simulink model "robot_1"  (R2016a)
settings: Solver=ode1  StartTime=0.0  StopTime=1000  FixedStep=0.05  RelTol=1e-3
undefined symbols (not defined in the file): Angular, Linear
libraries: robotlib x4, realtime_pacer_lib x2, simulink x2
settings Model: Creator=Esther  LastModifiedBy=Esther
settings DataIOCC: LimitDataPoints=on  SaveFormat=Array
settings OptimizationCC: OptimizeModelRefInitCode=on  LifeSpan=1  MaxStackSize=64
settings HardwareCC: ProdBitPerPointer=32  ProdLargestAtomicFloat=None  ProdIntDivRoundTo=Undefined  ProdEndianess=Unspecified  ProdWordSize=32  ProdHWDeviceType=Generic->Unspecified (assume 32-bit Generic)
settings ModelReferenceCC: PropagateSignalLabelsOutOfModel=off
settings RTWCC: SystemTargetFile=ert.tlc  HardwareBoard=Robot Operating System (ROS)  PackageName=robot_1  TemplateMakefile=ert_default_tmf  Toolchain=Catkin  TargetLang=C++
settings ERTTargetCC: SupportContinuousTime=on  SupportVariableSizeSignals=on  RootIOFormat=Structure reference  ConvertIfToSwitch=off  SuppressUnreachableDefaultCases=off
settings ConfigComp: CovModelRefEnable=Off

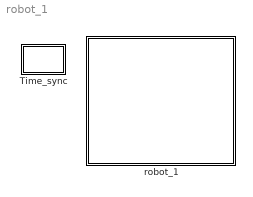
== system robot_1 ==
  Time_sync : Subsystem
  robot_1 : Subsystem

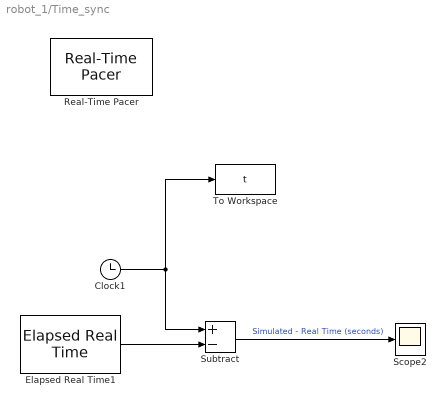
== system robot_1/Time_sync ==
  Clock1 : Clock
  Elapsed Real Time1 : realtime_pacer_lib/Elapsed Real Time
  Real-Time Pacer : realtime_pacer_lib/Real-Time Pacer  simTimePerRealTime=1
  Scope2 : Scope
  Subtract : Sum  Inputs=+-
  To Workspace : ToWorkspace  VariableName=t  SampleTime=-1
  wires:
  Elapsed Real Time1/1 -> Subtract/2
  Subtract/1 -> Scope2/1  "Simulated - Real Time (seconds)"
  Clock1/1 -> To Workspace/1, Subtract/1

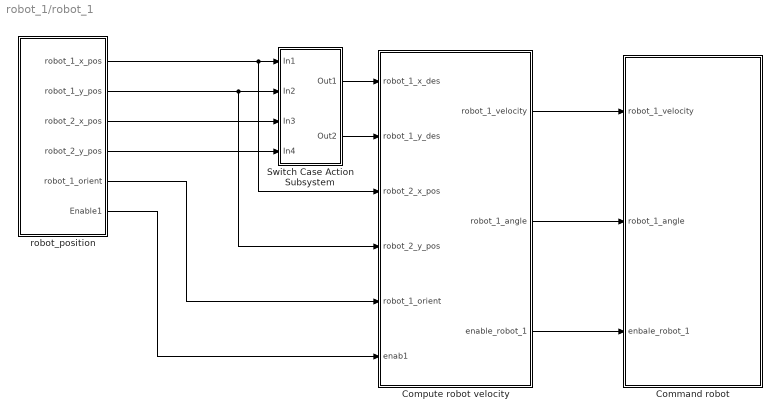
== system robot_1/robot_1 ==
  Command robot : Subsystem
  Compute robot velocity : Subsystem
  Switch Case Action Subsystem : Subsystem  TreatAsAtomicUnit=on
  robot_position : Subsystem
  wires:
  Compute robot velocity/1(robot_1_velocity) -> Command robot/1(robot_1_velocity)
  Compute robot velocity/3(enable_robot_1) -> Command robot/3(enbale_robot_1)
  robot_position/6(Enable1) -> Compute robot velocity/6(enab1)
  Switch Case Action Subsystem/1(Out1) -> Compute robot velocity/1(robot_1_x_des)
  robot_position/3(robot_2_x_pos) -> Switch Case Action Subsystem/3(In3)
  Switch Case Action Subsystem/2(Out2) -> Compute robot velocity/2(robot_1_y_des)
  robot_position/4(robot_2_y_pos) -> Switch Case Action Subsystem/4(In4)
  Compute robot velocity/2(robot_1_angle) -> Command robot/2(robot_1_angle)
  robot_position/5(robot_1_orient) -> Compute robot velocity/5(robot_1_orient)
  robot_position/2(robot_1_y_pos) -> Compute robot velocity/4(robot_2_y_pos), Switch Case Action Subsystem/2(In2)
  robot_position/1(robot_1_x_pos) -> Compute robot velocity/3(robot_2_x_pos), Switch Case Action Subsystem/1(In1)

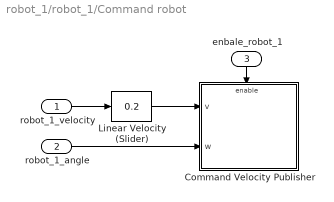
== system robot_1/robot_1/Command robot ==
  robot_1_velocity : Inport
  robot_1_angle : Inport  Port=2
  enbale_robot_1 : Inport  Port=3
  Command Velocity Publisher : Subsystem
  Linear Velocity (Slider) : simulink/Math Operations/Slider Gain  low=0  gain=0.2  high=1
  wires:
  robot_1_angle/1 -> Command Velocity Publisher/2(w)
  enbale_robot_1/1 -> Command Velocity Publisher/Enable
  robot_1_velocity/1 -> Linear Velocity (Slider)/1
  Linear Velocity (Slider)/1 -> Command Velocity Publisher/1(v)

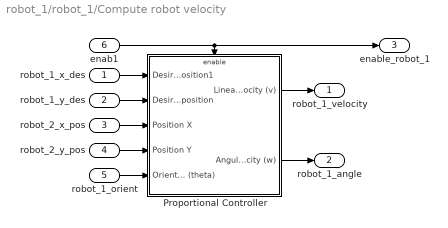
== system robot_1/robot_1/Compute robot velocity ==
  robot_1_x_des : Inport
  robot_1_y_des : Inport  Port=2
  robot_2_x_pos : Inport  Port=3
  robot_2_y_pos : Inport  Port=4
  robot_1_orient : Inport  Port=5
  enab1 : Inport  Port=6
  Proportional Controller : Subsystem
  robot_1_velocity : Outport
  robot_1_angle : Outport  Port=2
  enable_robot_1 : Outport  Port=3
  wires:
  Proportional Controller/1(Linear Velocity (v)) -> robot_1_velocity/1
  Proportional Controller/2(Angular Velocity (w)) -> robot_1_angle/1
  robot_2_x_pos/1 -> Proportional Controller/3(Position X)
  robot_1_orient/1 -> Proportional Controller/5(Orientation (theta))
  robot_1_x_des/1 -> Proportional Controller/1(Desired position1)
  robot_2_y_pos/1 -> Proportional Controller/4(Position Y)
  robot_1_y_des/1 -> Proportional Controller/2(Desired position)
  enab1/1 -> enable_robot_1/1, Proportional Controller/Enable

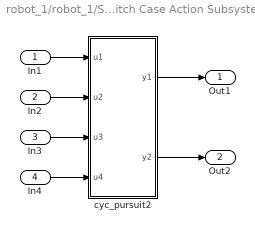
== system robot_1/robot_1/Switch Case Action Subsystem ==
  In1 : Inport
  In2 : Inport  Port=2
  In3 : Inport  Port=3
  In4 : Inport  Port=4
  cyc_pursuit2 : MATLAB Function  TreatAsAtomicUnit=on
  Out1 : Outport
  Out2 : Outport  Port=2
  wires:
  In4/1 -> cyc_pursuit2/4(u4)
  In3/1 -> cyc_pursuit2/3(u3)
  cyc_pursuit2/2(y2) -> Out2/1
  In2/1 -> cyc_pursuit2/2(u2)
  cyc_pursuit2/1(y1) -> Out1/1
  In1/1 -> cyc_pursuit2/1(u1)

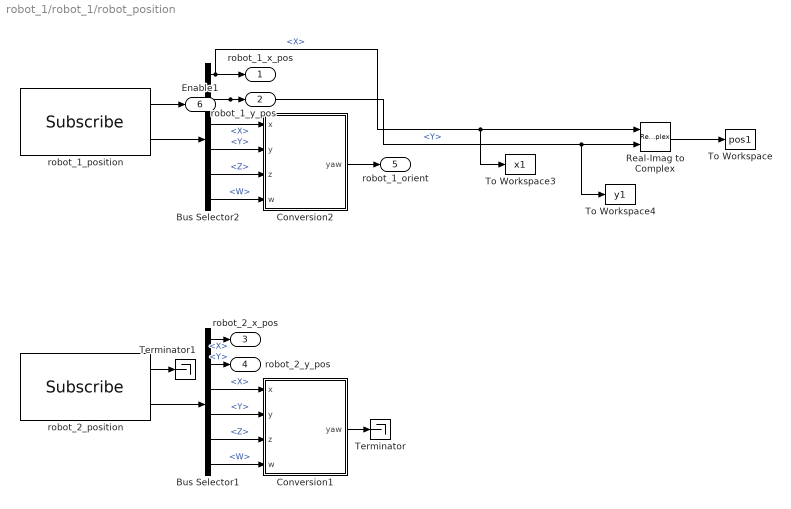
== system robot_1/robot_1/robot_position ==
  Bus Selector1 : BusSelector  OutputSignals=Pose.Pose.Position.X,Pose.Pose.Position.Y,Pose.Pose.Orientation.X,Pose.Pose.Orientation.Y,Pose.Pose.Orientation.Z,Pose.Pose.Orientation.W
  Bus Selector2 : BusSelector  OutputSignals=Pose.Pose.Position.X,Pose.Pose.Position.Y,Pose.Pose.Orientation.X,Pose.Pose.Orientation.Y,Pose.Pose.Orientation.Z,Pose.Pose.Orientation.W
  Conversion1 : MATLAB Function  TreatAsAtomicUnit=on
  Conversion2 : MATLAB Function  TreatAsAtomicUnit=on
  Real-Imag to Complex : RealImagToComplex
  Terminator : Terminator
  Terminator1 : Terminator
  To Workspace : ToWorkspace  VariableName=pos1  SampleTime=-1
  To Workspace3 : ToWorkspace  VariableName=x1  SampleTime=-1
  To Workspace4 : ToWorkspace  VariableName=y1  SampleTime=-1
  robot_1_position : robotlib/Subscribe  SourceLibraryInfo=This block requires Robotics System Toolbox  topicSource=Select from ROS network  topic=/robot_1/base_pose_ground_truth  messageType=nav_msgs/Odometry  sampleTime=-1  messageQueueLength=1
  robot_2_position : robotlib/Subscribe  SourceLibraryInfo=This block requires Robotics System Toolbox  topicSource=Select from ROS network  topic=/robot_2/base_pose_ground_truth  messageType=nav_msgs/Odometry  sampleTime=-1  messageQueueLength=1
  robot_1_x_pos : Outport
  robot_1_y_pos : Outport  Port=2
  robot_2_x_pos : Outport  Port=3
  robot_2_y_pos : Outport  Port=4
  robot_1_orient : Outport  Port=5
  Enable1 : Outport  Port=6
  wires:
  Bus Selector2/5 -> Conversion2/3(z)  "<Z>"
  robot_1_position/1 -> Enable1/1
  Bus Selector2/1 -> robot_1_x_pos/1, To Workspace3/1, Real-Imag to Complex/1  "<X>"
  Bus Selector2/4 -> Conversion2/2(y)  "<Y>"
  Bus Selector2/3 -> Conversion2/1(x)  "<X>"
  Real-Imag to Complex/1 -> To Workspace/1
  Bus Selector2/6 -> Conversion2/4(w)  "<W>"
  Bus Selector2/2 -> robot_1_y_pos/1, To Workspace4/1, Real-Imag to Complex/2  "<Y>"
  robot_1_position/2 -> Bus Selector2/1
  Conversion2/1(yaw) -> robot_1_orient/1
  Conversion1/1(yaw) -> Terminator/1
  Bus Selector1/1 -> robot_2_x_pos/1  "<X>"
  Bus Selector1/2 -> robot_2_y_pos/1  "<Y>"
  Bus Selector1/3 -> Conversion1/1(x)  "<X>"
  Bus Selector1/4 -> Conversion1/2(y)  "<Y>"
  Bus Selector1/5 -> Conversion1/3(z)  "<Z>"
  robot_2_position/2 -> Bus Selector1/1
  Bus Selector1/6 -> Conversion1/4(w)  "<W>"
  robot_2_position/1 -> Terminator1/1

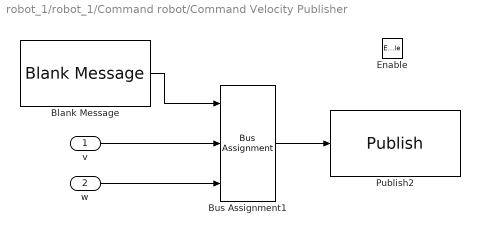
== system robot_1/robot_1/Command robot/Command Velocity Publisher ==
  v : Inport
  w : Inport  Port=2
  Enable : EnablePort
  Blank Message : robotlib/Blank Message  SourceLibraryInfo=This block requires Robotics System Toolbox  messageType=geometry_msgs/Twist  SampleTime=inf
  Bus Assignment1 : BusAssignment  DialogController=Simulink.DDGSource_BusAssignment  AssignedSignals=Linear.X,Angular.Z
  Publish2 : robotlib/Publish  SourceLibraryInfo=This block requires Robotics System Toolbox  topicSource=Select from ROS network  topic=/robot_1/cmd_vel  messageType=geometry_msgs/Twist  messageQueueLength=105
  wires:
  Bus Assignment1/1 -> Publish2/1
  Blank Message/1 -> Bus Assignment1/1
  v/1 -> Bus Assignment1/2
  w/1 -> Bus Assignment1/3

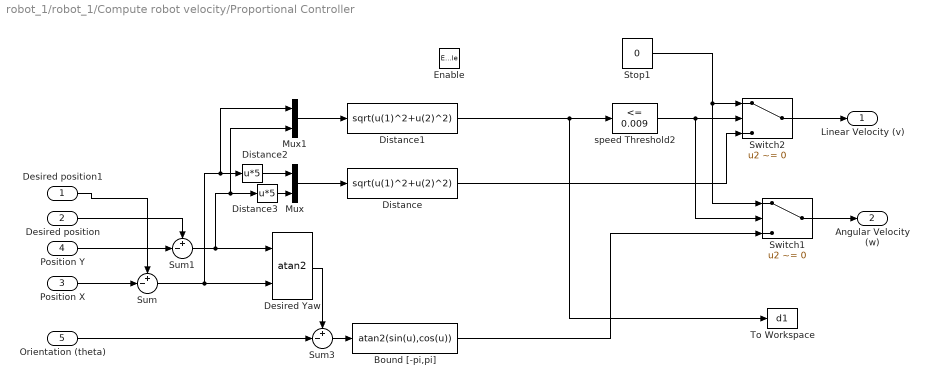
== system robot_1/robot_1/Compute robot velocity/Proportional Controller ==
  Desired position1 : Inport
  Desired position : Inport  Port=2
  Position X : Inport  Port=3
  Position Y : Inport  Port=4
  Orientation (theta) : Inport  Port=5
  Enable : EnablePort
  Bound [-pi,pi] : Fcn  Expr=atan2(sin(u),cos(u))
  Desired Yaw : Trigonometry  Operator=atan2
  Distance : Fcn  Expr=sqrt(u(1)^2+u(2)^2)
  Distance1 : Fcn  Expr=sqrt(u(1)^2+u(2)^2)
  Distance2 : Fcn  Expr=u*5
  Distance3 : Fcn  Expr=u*5
  Mux : Mux  Inputs=2
  Mux1 : Mux  Inputs=2
  Stop1 : Constant  Value=0
  Sum : Sum  Inputs=+-|
  Sum1 : Sum  Inputs=+-|
  Sum3 : Sum  Inputs=+-|
  Switch1 : Switch  Criteria=u2 ~= 0
  Switch2 : Switch  Criteria=u2 ~= 0
  To Workspace : ToWorkspace  VariableName=d1  SampleTime=-1
  speed Threshold2 : simulink/Logic and Bit Operations/Compare To Constant  relop=<=  const=0.009  OutDataTypeStr=boolean
  Linear Velocity (v) : Outport
  Angular Velocity (w) : Outport  Port=2
  wires:
  Desired position1/1 -> Sum/1
  Desired position/1 -> Sum1/1
  Position Y/1 -> Sum1/2
  Position X/1 -> Sum/2
  Mux/1 -> Distance/1
  Orientation (theta)/1 -> Sum3/2
  Desired Yaw/1 -> Sum3/1
  Sum3/1 -> Bound [-pi,pi]/1
  Distance/1 -> Switch2/3
  Distance2/1 -> Mux/1
  Distance3/1 -> Mux/2
  Mux1/1 -> Distance1/1
  Sum/1 -> Desired Yaw/2, Mux1/1, Distance2/1
  Sum1/1 -> Desired Yaw/1, Mux1/2, Distance3/1
  speed Threshold2/1 -> Switch2/2, Switch1/2
  Bound [-pi,pi]/1 -> Switch1/3
  Stop1/1 -> Switch2/1, Switch1/1
  Distance1/1 -> To Workspace/1, speed Threshold2/1
  Switch1/1 -> Angular Velocity (w)/1
  Switch2/1 -> Linear Velocity (v)/1

== matlab function robot_1/Switch Case Action Subsystem/cyc_pursuit2 ==
  data: u1 input; y1 output; u2 input; u3 input; u4 input; y2 output
function [y1, y2] = fcn(u1, u2, u3, u4)
%#codegen


y1 = ((1-0.2)*u1+(u3*0.2)-(2.5000*0.2));
y2 = ((1-0.2)*u2+(0.2*u4)-(4.33012*0.2));

== matlab function robot_1/robot_position/Conversion1 ==
  data: yaw output; x input; y input; z input; w input
function yaw  = quat2eul(x,y,z,w)
%#codegen

% Convert the quaternion to a yaw angle (zyx euler angle)
eul = quat2eul([w,x,y,z]);
yaw = eul(1);

end

== matlab function robot_1/robot_position/Conversion2 ==
  data: yaw output; x input; y input; z input; w input
function yaw  = quat2eul(x,y,z,w)
%#codegen

% Convert the quaternion to a yaw angle (zyx euler angle)
eul = quat2eul([w,x,y,z]);
yaw = eul(1);

end
